simulink model "BPSK_BER1"  (Simulink 6.5)
settings: Solver=VariableStepDiscrete  StartTime=0.0  StopTime=10.0  RelTol=1e-3
values from neighbouring files (symbols this model uses):
  xSampleTime = 1/100000    (= 1e-05)    [Simulink_BPSK_BER.m]    (also in Simulink_BSC_BER.m)
libraries: commdigbbndpm3 x2, commchan3 x1, commsink2 x1, commrandsrc2 x1
settings Model: Creator=Administrator  LastModifiedBy=Administrator

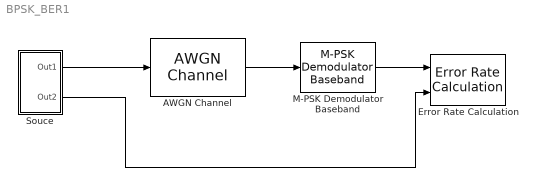
== system BPSK_BER1 ==
  AWGN Channel : commchan3/AWGN Channel  SystemSampleTime=-1  seed=xInitialSeed  noiseMode="Signal to noise ratio  (SNR)"  EbNodB=xSNR  EsNodB=10  SNRdB=xSNR  bitsPerSym=1  Ps=1  Tsym=1  variance=1
  Error Rate Calculation : commsink2/Error Rate Calculation  N=0  st_delay=0  cp_mode=Entire frame  subframe=[]  PMode=Workspace  WsName=xErrorRate  RsMode2=off  stop=off  numErr=100  maxBits=1e6
  M-PSK Demodulator Baseband : commdigbbndpm3/M-PSK Demodulator Baseband  DialogController=commDDGCreate  DialogControllerArgs=DataTag0  M=2  Ph=pi/2  Dec=Binary  Mapping=[0:7]  OutType=Bit  DecType=Hard decision  VarSource=Dialog  Variance=1  outDtype1=double  outDtype2=double
  Souce : Subsystem
  wires:
  Souce/1(Out1) -> AWGN Channel/1
  Souce/2(Out2) -> Error Rate Calculation/2
  AWGN Channel/1 -> M-PSK Demodulator Baseband/1
  M-PSK Demodulator Baseband/1 -> Error Rate Calculation/1

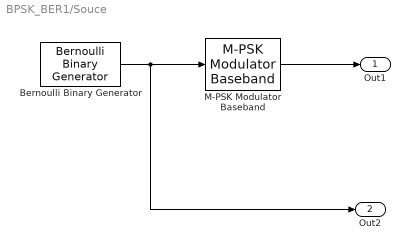
== system BPSK_BER1/Souce ==
  Bernoulli Binary Generator : commrandsrc2/Bernoulli Binary Generator  DialogController=commDDGCreate  DialogControllerArgs=DataTag1  SystemSampleTime=-1  P=0.5  seed=xInitialSeed  Ts=xSampleTime  frameBased=on  sampPerFrame=1  orient=off  outDataType=double
  M-PSK Modulator Baseband : commdigbbndpm3/M-PSK Modulator Baseband  M=2  InType=Bit  Enc=Binary  Mapping=0  Ph=pi/2  outDtype=double  outWordLen=16  outUDDataType=sfix(16)  outFracLenMode=Best precision  outFracLen=15
  Out1 : Outport
  Out2 : Outport  Port=2
  wires:
  Bernoulli Binary Generator/1 -> M-PSK Modulator Baseband/1, Out2/1
  M-PSK Modulator Baseband/1 -> Out1/1
